simulink model "mloc_sens_vloc"  (R2018b)
settings: configuration reference "Active" (kept outside this file)
undefined symbols (not defined in the file): TUMHealthStatus
libraries: simulink x3, rr_general x1
settings Model: DataDictionary=mloc_sens_vloc.sldd  Creator=wischnewski  LastModifiedBy=ge34qer

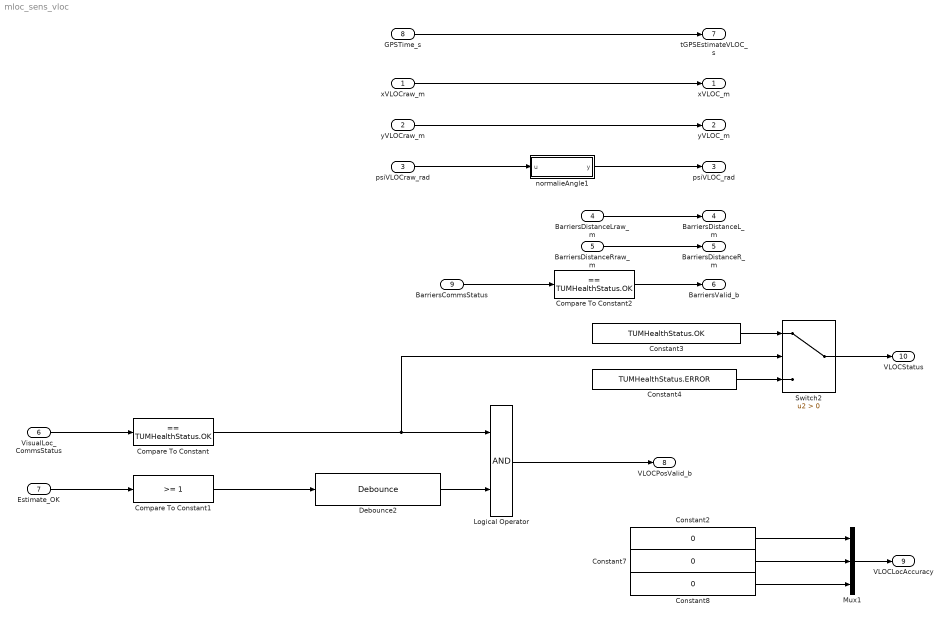
== system mloc_sens_vloc ==
  xVLOCraw_m : Inport
  yVLOCraw_m : Inport  Port=2
  "psiVLOCraw_rad " : Inport  Port=3
  BarriersDistanceLraw_m : Inport  Port=4
  BarriersDistanceRraw_m : Inport  Port=5
  VisualLoc_CommsStatus : Inport  Port=6  OutDataTypeStr=Enum: TUMHealthStatus
  Estimate_OK : Inport  Port=7  OutDataTypeStr=uint16
  GPSTime_s : Inport  Port=8
  BarriersCommsStatus : Inport  Port=9  OutDataTypeStr=Enum: TUMHealthStatus
  Compare To Constant : simulink/Logic and Bit Operations/Compare To Constant  relop===  const=TUMHealthStatus.OK  OutDataTypeStr=boolean
  Compare To Constant1 : simulink/Logic and Bit Operations/Compare To Constant  relop=>=  const=1  OutDataTypeStr=boolean
  Compare To Constant2 : simulink/Logic and Bit Operations/Compare To Constant  relop===  const=TUMHealthStatus.OK  OutDataTypeStr=boolean
  Constant2 : Constant  Value=0
  Constant3 : Constant  Value=TUMHealthStatus.OK  OutDataTypeStr=Enum: TUMHealthStatus
  Constant4 : Constant  Value=TUMHealthStatus.ERROR  OutDataTypeStr=Enum: TUMHealthStatus
  Constant7 : Constant  Value=0
  Constant8 : Constant  Value=0
  Debounce2 : rr_general/Debounce  debounce_cycles=P_MLOC_DebounceVLOC
  Logical Operator : Logic  AllPortsSameDT=off  OutDataTypeStr=boolean
  Mux1 : Mux  Inputs=3
  Switch2 : Switch  Criteria=u2 > Threshold
  normalieAngle1 : MATLAB Function  TreatAsAtomicUnit=on
  xVLOC_m : Outport
  yVLOC_m : Outport  Port=2
  psiVLOC_rad : Outport  Port=3
  BarriersDistanceL_m : Outport  Port=4
  BarriersDistanceR_m : Outport  Port=5
  BarriersValid_b : Outport  Port=6  OutDataTypeStr=boolean
  tGPSEstimateVLOC_s : Outport  Port=7
  VLOCPosValid_b : Outport  Port=8  OutDataTypeStr=boolean
  VLOCLocAccuracy : Outport  Port=9
  VLOCStatus : Outport  Port=10  OutDataTypeStr=Enum: TUMHealthStatus
  wires:
  GPSTime_s/1 -> tGPSEstimateVLOC_s/1
  VisualLoc_CommsStatus/1 -> Compare To Constant/1
  Constant4/1 -> Switch2/3
  Constant3/1 -> Switch2/1
  Switch2/1 -> VLOCStatus/1
  Logical Operator/1 -> VLOCPosValid_b/1
  Compare To Constant1/1 -> Debounce2/1
  Estimate_OK/1 -> Compare To Constant1/1
  Debounce2/1 -> Logical Operator/2
  BarriersDistanceLraw_m/1 -> BarriersDistanceL_m/1
  BarriersDistanceRraw_m/1 -> BarriersDistanceR_m/1
  yVLOCraw_m/1 -> yVLOC_m/1
  xVLOCraw_m/1 -> xVLOC_m/1
  Compare To Constant/1 -> Switch2/2, Logical Operator/1
  "psiVLOCraw_rad "/1 -> normalieAngle1/1(u)
  normalieAngle1/1(y) -> psiVLOC_rad/1
  BarriersCommsStatus/1 -> Compare To Constant2/1
  Compare To Constant2/1 -> BarriersValid_b/1
  Constant7/1 -> Mux1/2
  Constant2/1 -> Mux1/1
  Mux1/1 -> VLOCLocAccuracy/1
  Constant8/1 -> Mux1/3

== matlab function mloc_sens_vloc/normalieAngle1 ==
  data: u input; y output
function y = fcn(u)

y = normalizeAngle(u);
